simulink model "detect_fall_simu"  (Simulink 8.4)
settings: Solver=VariableStepDiscrete  StartTime=0.0  StopTime=1  MaxStep=1  RelTol=1e-3
libraries: simulink x2
settings Model: Creator=arnaud  LastModifiedBy=arnaud
settings DataIOCC: SaveFormat=Structure  SignalLoggingSaveFormat=Dataset
settings OptimizationCC: ExpressionDepthLimit=128
settings DebuggingCC: UnderspecifiedInitializationDetection=Simplified  MergeDetectMultiDrivingBlocksExec=error  FcnCallInpInsideContextMsg=EnableAllAsError  StateNameClashWarn=none
settings GRTTargetCC: CombineOutputUpdateFcns=on  GRTInterface=off

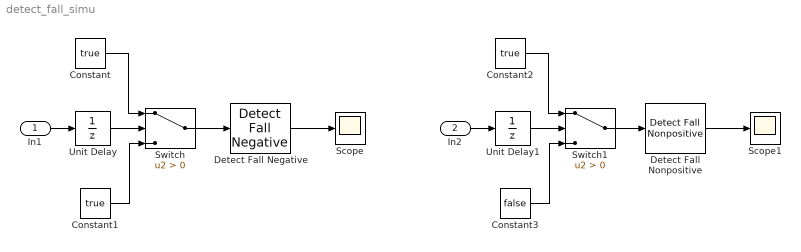
== system detect_fall_simu ==
  In1 : Inport
  In2 : Inport  Port=2
  Constant : Constant  Value=true
  Constant1 : Constant  Value=true
  Constant2 : Constant  Value=true
  Constant3 : Constant  Value=false
  Detect Fall Negative : simulink/Logic and Bit Operations/Detect Fall Negative  vinit=0  InputProcessing=Inherited  OutDataTypeStr=boolean
  Detect Fall Nonpositive : simulink/Logic and Bit Operations/Detect Fall Nonpositive  vinit=0  InputProcessing=Inherited  OutDataTypeStr=boolean
  Scope : Scope
  Scope1 : Scope
  Switch : Switch  Criteria=u2 > Threshold
  Switch1 : Switch  Criteria=u2 > Threshold
  Unit Delay : UnitDelay  InitialCondition=1  SampleTime=-1
  Unit Delay1 : UnitDelay  InitialCondition=1  SampleTime=-1
  wires:
  Detect Fall Negative/1 -> Scope/1
  In1/1 -> Unit Delay/1
  Unit Delay/1 -> Switch/2
  Constant/1 -> Switch/1
  Constant1/1 -> Switch/3
  Switch/1 -> Detect Fall Negative/1
  In2/1 -> Unit Delay1/1
  Unit Delay1/1 -> Switch1/2
  Constant2/1 -> Switch1/1
  Constant3/1 -> Switch1/3
  Switch1/1 -> Detect Fall Nonpositive/1
  Detect Fall Nonpositive/1 -> Scope1/1
